simulink model "hetau"  (R2020b)
settings: Solver=VariableStepAuto  StartTime=0.0  StopTime=10.0  RelTol=1e-3
settings Model: Creator=ACER  LastModifiedBy=ACER

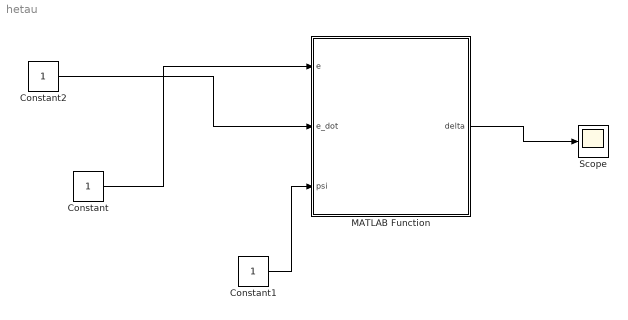
== system hetau ==
  Constant : Constant
  Constant1 : Constant
  Constant2 : Constant
  MATLAB Function : MATLAB Function  TreatAsAtomicUnit=on
  Scope : Scope
  wires:
  Constant2/1 -> MATLAB Function/2(e_dot)
  Constant/1 -> MATLAB Function/1(e)
  Constant1/1 -> MATLAB Function/3(psi)
  MATLAB Function/1(delta) -> Scope/1

== matlab function hetau/MATLAB Function ==
  data: e input; delta output; e_dot input; psi input
function delta = fcn(e, e_dot, psi)
l = 161;
v=5;
k0=-3.86;
tau10 =5.66;
tau20 =0.38;
tau30 =0.89;
k=k0*(v/l);
tau1 = tau10* (l/v);
tau2 = tau20* (l/v);
tau3 = tau30* (l/v);
psi_3dot = (k/(tau1*tau2))*(tau3*delta_dot+delta)-((1/tau3)+(1/tau2))*psi_3dot+(1/tau1*tau2)*(psi_dot^3+psi_dot)
psi_3dot = u;
